simulink model "Full_state_feeback_control_model"  (R2021a)
settings: Solver=VariableStepAuto  StartTime=0.0  StopTime=10.0  RelTol=1e-3
values from neighbouring files (symbols this model uses):
  A = [0 1 0 0 ... (first row only)    [Controllability_of_a_Linear_System.m]    (also in Full_State_Feedback_Control_Design.m = [0 3;2 4]; Implementation_Issues_with_a_FSFB.m = [0 1 0; Introduction_to_Full_State_Feedback_COntrol.m = [0 3;2 4]; Introduction_to_LQR_control.m = [0 1)
  B = [0 ... (first row only)    [Controllability_of_a_Linear_System.m]    (also in Full_State_Feedback_Control_Design.m = [-2 1; 1 1]; Implementation_Issues_with_a_FSFB.m = [0 0; Introduction_to_Full_State_Feedback_COntrol.m = [-2 1; 1 1]; Introduction_to_LQR_control.m)
  C = eye(3)    [Implementation_Issues_with_a_FSFB.m]    (also in Kalman_Filter_Design.m = [1 0 0 0]; Observability_example.m = [1 0 0 1]; Observability_gramion_example.m = [0 0 1]; Practical_Implementation_Issues_with_a_FSFB.m)
  D = zeros(3,2)    [Implementation_Issues_with_a_FSFB.m]    (also in Kalman_Filter_Design.m = zeros(size(C,1),size(B,1)); Observability_gramion_example.m = zeros(1,size(B,2)))
  K = place(A,B(:,1),desired_closed_loop_poles)    [Implementation_Issues_with_a_FSFB.m]    (also in Practical_Implementation_Issues_with_a_FSFB.m)
  x0 = [72*pi/180 ... (first row only)    [Implementation_Issues_with_a_FSFB.m]    (also in Introduction_to_LQR_control.m = [pi; LQR_control.m = [pi)
settings Model: Creator=subhi  LastModifiedBy=subhi

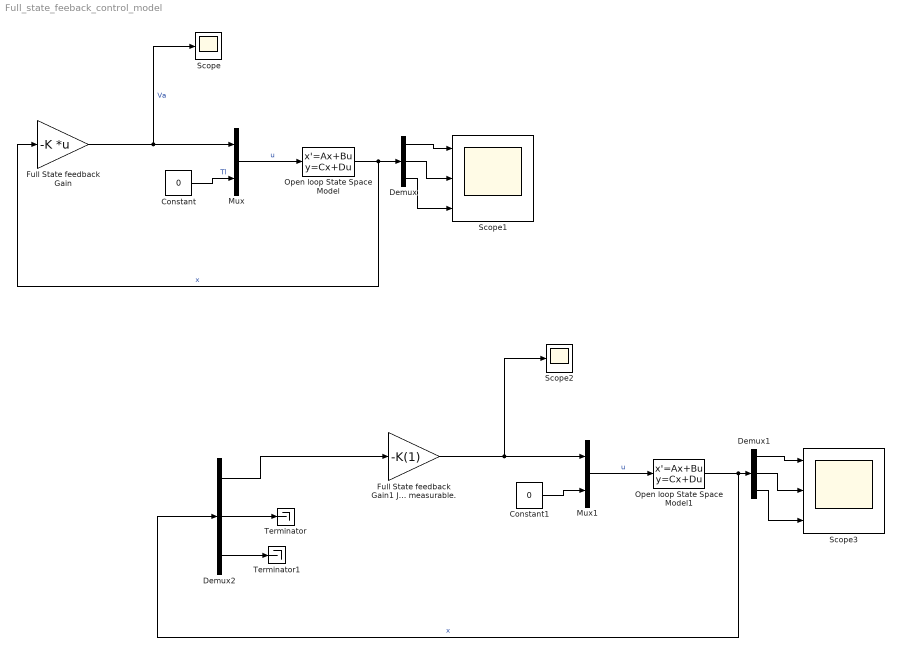
== system Full_state_feeback_control_model ==
  Constant : Constant  Value=0
  Constant1 : Constant  Value=0
  Demux : Demux  Outputs=3
  Demux1 : Demux  Outputs=3
  Demux2 : Demux  Outputs=3
  Full State feedback Gain1 Just changing the poles for the states are measurable. : Gain  Gain=-K(1)
  Full State feedback Gain : Gain  Gain=-K  Multiplication=Matrix(K*u)
  Mux : Mux  Inputs=2
  Mux1 : Mux  Inputs=2
  Open loop State Space Model : StateSpace  A=A  B=B  C=C  D=D  InitialCondition=x0
  Open loop State Space Model1 : StateSpace  A=A  B=B  C=C  D=D  InitialCondition=x0
  Scope : Scope
  Scope1 : Scope  NumInputPorts=3
  Scope2 : Scope
  Scope3 : Scope  NumInputPorts=3
  Terminator : Terminator
  Terminator1 : Terminator
  wires:
  Open loop State Space Model/1 -> Demux/1, Full State feedback Gain/1  "x"
  Full State feedback Gain/1 -> Scope/1, Mux/1  "Va"
  Mux/1 -> Open loop State Space Model/1  "u"
  Constant/1 -> Mux/2  "Tl"
  Demux/2 -> Scope1/2
  Demux/1 -> Scope1/1
  Demux/3 -> Scope1/3
  Mux1/1 -> Open loop State Space Model1/1  "u"
  Constant1/1 -> Mux1/2
  Demux1/1 -> Scope3/1
  Demux1/2 -> Scope3/2
  Open loop State Space Model1/1 -> Demux2/1, Demux1/1  "x"
  Demux1/3 -> Scope3/3
  Full State feedback Gain1 Just changing the poles for the states are measurable./1 -> Scope2/1, Mux1/1
  Demux2/1 -> Full State feedback Gain1 Just changing the poles for the states are measurable./1
  Demux2/2 -> Terminator/1
  Demux2/3 -> Terminator1/1
